simulink model "Tracking"  (R2016a)
settings: Solver=VariableStepAuto  StartTime=0.0  StopTime=20  RelTol=1e-3
undefined symbols (not defined in the file): L1, L12, L2
settings Model: Creator=UTM_Hugo  LastModifiedBy=UTM_Hugo

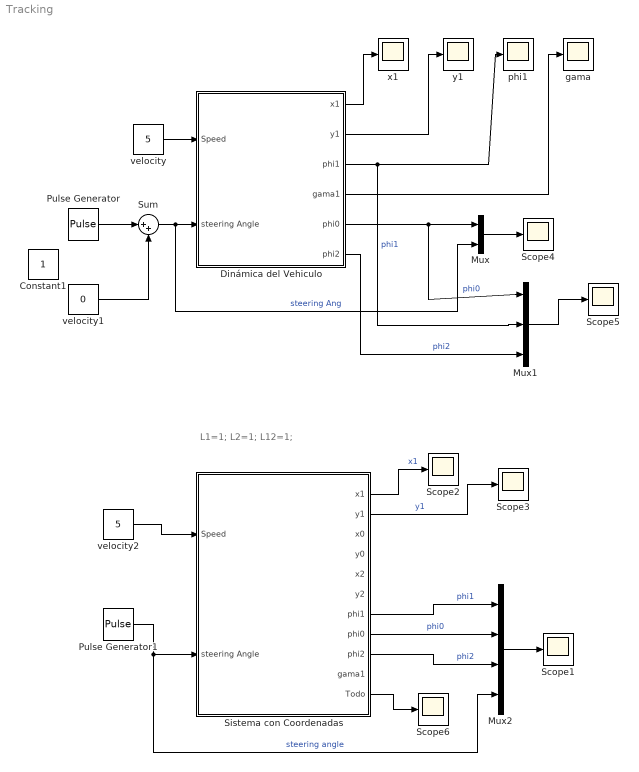
== system Tracking ==
  note: L1=1; L2=1; L12=1;
  Constant1 : Constant
  Dinámica del Vehiculo : Subsystem
  Mux : Mux  Inputs=2
  Mux1 : Mux  Inputs=3
  Mux2 : Mux
  Pulse Generator : DiscretePulseGenerator  PulseType=Time based  Amplitude=0.1  Period=10  PulseWidth=5
  Pulse Generator1 : DiscretePulseGenerator  PulseType=Time based  Amplitude=0.1  Period=10  PulseWidth=5
  Scope{1..6} (6 alike) : Scope
  Sistema con Coordenadas : Subsystem
  Sum : Sum  Inputs=|++
  gama : Scope
  phi1 : Scope
  velocity : Constant  Value=5
  velocity1 : Constant  Value=0
  velocity2 : Constant  Value=5
  x1 : Scope
  y1 : Scope
  wires:
  velocity/1 -> Dinámica del Vehiculo/1(Speed)
  Dinámica del Vehiculo/1(x1) -> x1/1
  Dinámica del Vehiculo/2(y1) -> y1/1
  Dinámica del Vehiculo/3(phi1) -> phi1/1, Mux1/2  "phi1"
  Dinámica del Vehiculo/4(gama1) -> gama/1
  Dinámica del Vehiculo/5(phi0) -> Mux1/1, Mux/1  "phi0"
  Mux/1 -> Scope4/1
  Pulse Generator/1 -> Sum/1
  Sum/1 -> Mux/2, Dinámica del Vehiculo/2(steering Angle)  "steering Ang"
  velocity1/1 -> Sum/2
  Mux1/1 -> Scope5/1
  Dinámica del Vehiculo/6(phi2) -> Mux1/3  "phi2"
  Pulse Generator1/1 -> Mux2/4, Sistema con Coordenadas/2(steering Angle)  "steering angle"
  velocity2/1 -> Sistema con Coordenadas/1(Speed)
  Sistema con Coordenadas/7(phi1) -> Mux2/1  "phi1"
  Sistema con Coordenadas/8(phi0) -> Mux2/2  "phi0"
  Sistema con Coordenadas/9(phi2) -> Mux2/3  "phi2"
  Mux2/1 -> Scope1/1
  Sistema con Coordenadas/1(x1) -> Scope2/1  "x1"
  Sistema con Coordenadas/2(y1) -> Scope3/1  "y1"
  Sistema con Coordenadas/11(Todo) -> Scope6/1

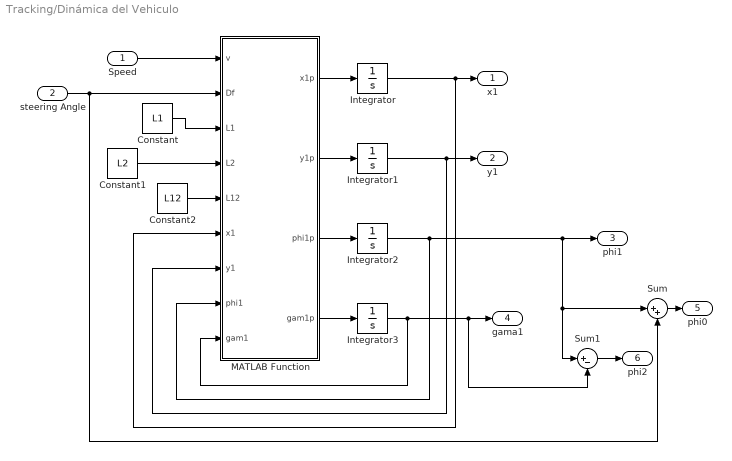
== system Tracking/Dinámica del Vehiculo ==
  Speed : Inport
  steering Angle : Inport  Port=2
  Constant : Constant  Value=L1
  Constant1 : Constant  Value=L2
  Constant2 : Constant  Value=L12
  Integrator{,1..3} (4 alike) : Integrator
  MATLAB Function : MATLAB Function  TreatAsAtomicUnit=on
  Sum : Sum  Inputs=|++
  Sum1 : Sum  Inputs=|+-
  x1 : Outport
  y1 : Outport  Port=2
  phi1 : Outport  Port=3
  gama1 : Outport  Port=4
  phi0 : Outport  Port=5
  phi2 : Outport  Port=6
  wires:
  MATLAB Function/4(gam1p) -> Integrator3/1
  MATLAB Function/1(x1p) -> Integrator/1
  Speed/1 -> MATLAB Function/1(v)
  steering Angle/1 -> Sum/2, MATLAB Function/2(Df)
  Integrator3/1 -> MATLAB Function/9(gam1), Sum1/2, gama1/1
  MATLAB Function/3(phi1p) -> Integrator2/1
  MATLAB Function/2(y1p) -> Integrator1/1
  Integrator2/1 -> MATLAB Function/8(phi1), Sum1/1, Sum/1, phi1/1
  Integrator1/1 -> MATLAB Function/7(y1), y1/1
  Integrator/1 -> MATLAB Function/6(x1), x1/1
  Sum/1 -> phi0/1
  Constant/1 -> MATLAB Function/3(L1)
  Constant1/1 -> MATLAB Function/4(L2)
  Constant2/1 -> MATLAB Function/5(L12)
  Sum1/1 -> phi2/1

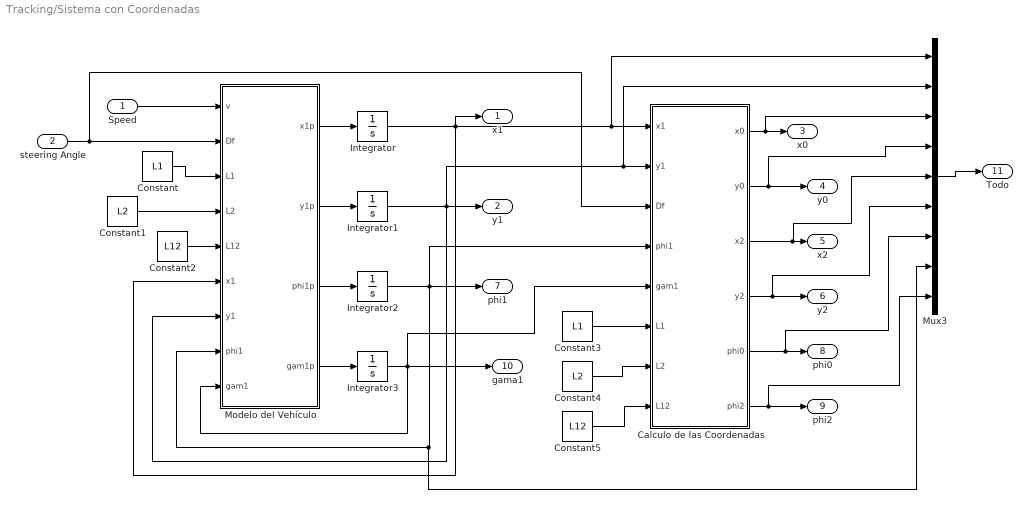
== system Tracking/Sistema con Coordenadas ==
  Speed : Inport
  steering Angle : Inport  Port=2
  Calculo de las Coordenadas : MATLAB Function  TreatAsAtomicUnit=on
  Constant : Constant  Value=L1
  Constant1 : Constant  Value=L2
  Constant2 : Constant  Value=L12
  Constant3 : Constant  Value=L1
  Constant4 : Constant  Value=L2
  Constant5 : Constant  Value=L12
  Integrator{,1..3} (4 alike) : Integrator
  Modelo del Vehículo : MATLAB Function  TreatAsAtomicUnit=on
  Mux3 : Mux  Inputs=9
  x1 : Outport
  y1 : Outport  Port=2
  x0 : Outport  Port=3
  y0 : Outport  Port=4
  x2 : Outport  Port=5
  y2 : Outport  Port=6
  phi1 : Outport  Port=7
  phi0 : Outport  Port=8
  phi2 : Outport  Port=9
  gama1 : Outport  Port=10
  Todo : Outport  Port=11
  wires:
  Modelo del Vehículo/4(gam1p) -> Integrator3/1
  Modelo del Vehículo/1(x1p) -> Integrator/1
  Speed/1 -> Modelo del Vehículo/1(v)
  steering Angle/1 -> Calculo de las Coordenadas/3(Df), Modelo del Vehículo/2(Df)
  Modelo del Vehículo/3(phi1p) -> Integrator2/1
  Modelo del Vehículo/2(y1p) -> Integrator1/1
  Integrator2/1 -> Calculo de las Coordenadas/4(phi1), Mux3/8, Modelo del Vehículo/8(phi1), phi1/1
  Integrator1/1 -> Modelo del Vehículo/7(y1), y1/1, Mux3/2, Calculo de las Coordenadas/2(y1)
  Integrator/1 -> Modelo del Vehículo/6(x1), x1/1, Mux3/1, Calculo de las Coordenadas/1(x1)
  Constant/1 -> Modelo del Vehículo/3(L1)
  Constant1/1 -> Modelo del Vehículo/4(L2)
  Constant2/1 -> Modelo del Vehículo/5(L12)
  Integrator3/1 -> Calculo de las Coordenadas/5(gam1), Modelo del Vehículo/9(gam1), gama1/1
  Constant3/1 -> Calculo de las Coordenadas/6(L1)
  Constant4/1 -> Calculo de las Coordenadas/7(L2)
  Constant5/1 -> Calculo de las Coordenadas/8(L12)
  Calculo de las Coordenadas/1(x0) -> Mux3/3, x0/1
  Calculo de las Coordenadas/2(y0) -> Mux3/4, y0/1
  Calculo de las Coordenadas/3(x2) -> Mux3/5, x2/1
  Calculo de las Coordenadas/4(y2) -> Mux3/6, y2/1
  Calculo de las Coordenadas/5(phi0) -> Mux3/7, phi0/1
  Calculo de las Coordenadas/6(phi2) -> Mux3/9, phi2/1
  Mux3/1 -> Todo/1

== matlab function Tracking/Sistema con Coordenadas/Modelo del Vehículo ==
  data: v input; Df input; L1 input; L2 input; L12 input; x1 input; y1 input; phi1 input; gam1 input; x1p output; y1p output; phi1p output; gam1p output
function [x1p,y1p,phi1p,gam1p] = fcn(v,Df,L1,L2,L12,x1,y1,phi1,gam1)
x1p=v*cos(phi1);
y1p=v*sin(phi1);
phi1p=(v/L1)*tan(Df);
temp1=(v/L1)+v*L12*cos(gam1)/(L1*L2);
gam1p=temp1*tan(Df)-v*sin(gam1)/L2;

== matlab function Tracking/Dinámica del Vehiculo/MATLAB Function ==
  data: v input; Df input; L1 input; L2 input; L12 input; x1 input; y1 input; phi1 input; gam1 input; x1p output; y1p output; phi1p output; gam1p output
function [x1p,y1p,phi1p,gam1p] = fcn(v,Df,L1,L2,L12,x1,y1,phi1,gam1)
x1p=v*cos(phi1);
y1p=v*sin(phi1);
phi1p=(v/L1)*tan(Df);
temp1=(v/L1)+v*L12*cos(gam1)/(L1*L2);
gam1p=temp1*tan(Df)-v*sin(gam1)/L2;

== matlab function Tracking/Sistema con Coordenadas/Calculo de las Coordenadas ==
  data: x1 input; y1 input; Df input; phi1 input; gam1 input; L1 input; L2 input; L12 input; x0 output; y0 output; x2 output; y2 output; phi0 output; phi2 output
function [x0,y0,x2,y2,phi0,phi2] = fcn(x1,y1,Df,phi1,gam1,L1,L2,L12)
phi2=phi1-gam1;
phi0=phi1+Df
x0=x1+L1*cos(phi1);
y0=y1+L1*sin(phi1);

x2=x1+L12*cos(phi1)+L2*cos(phi2);
y2=y1+L12*sin(phi1)+L2*sin(phi2);
